simulink model "HW7_simulink"  (R2021b)
settings: Solver=ode4  StartTime=0.0  StopTime=5  FixedStep=.005  RelTol=1e-3
values from neighbouring files (symbols this model uses):
  A = [1 0; 3 -1]    [HW2.m]    (also in HW5.m = [0 -1; 1 -1]; HW6.m = [-1 0; 0 -2]; HW7.m = double(subs(A_sym,[x1;x2;x3;x4;u],[x_star;u_star])))
  B = [1; 0]    [HW5.m]    (also in HW6.m = [1; 3]; HW7.m = double(subs(B_sym,[x1;x2;x3;x4;u],[x_star;u_star])))
  C = eye(2)    [HW5.m]    (also in HW7.m = [1 0 0 0;0 0 1 0])
  D = zeros(2,1)    [HW5.m]    (also in HW7.m)
  g = 10    [HW7.m]
  K = round(time/Ts)    [HW5.m]    (also in HW7.m = acker(A,B,s_desired))
  L = place(A',C',s_obs_desired)'    [HW7.m]
  l = 1    [HW7.m]
  m = 1    [HW7.m]
  M = [4 2 1; 4 -2 1; 4 1 0]    [HW2.m]    (also in HW7.m = 10)
undefined symbols (not defined in the file or in its folder): magnitude
settings Model: Creator=17165  LastModifiedBy=17165

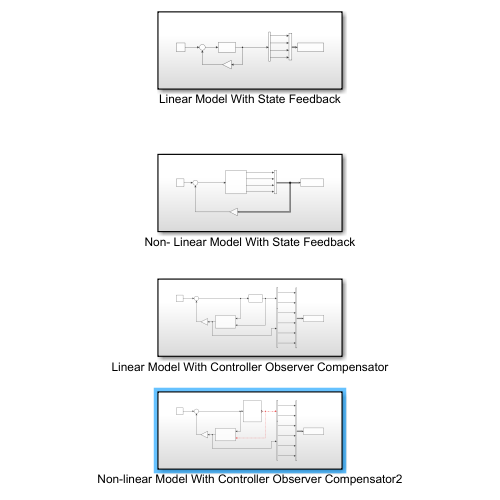
[thumbnail: Simulink's stored preview of the top-level diagram]
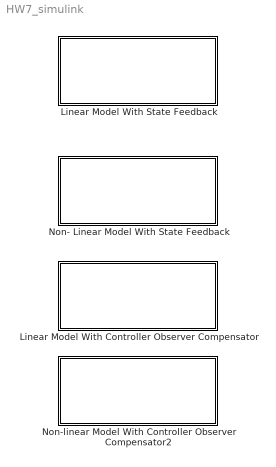
== system HW7_simulink ==
  Linear Model With Controller Observer Compensator : Subsystem
  Linear Model With State Feedback : Subsystem
  Non- Linear Model With State Feedback : Subsystem
  Non-linear Model With Controller Observer Compensator2 : Subsystem

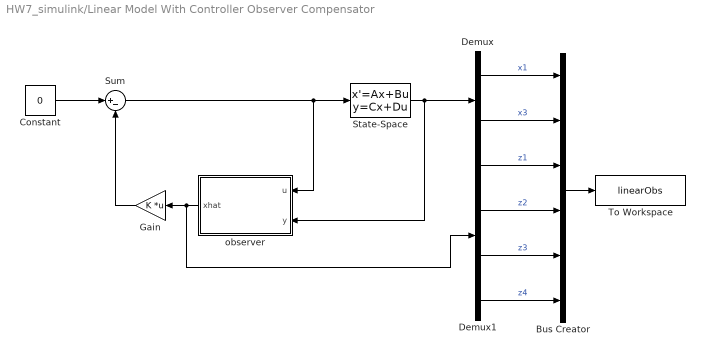
== system HW7_simulink/Linear Model With Controller Observer Compensator ==
  Bus Creator : BusCreator  Inputs=6
  Constant : Constant  Value=0
  Demux : Demux  Outputs=2
  Demux1 : Demux
  Gain : Gain  Gain=K  Multiplication=Matrix(K*u)
  State-Space : StateSpace  A=A  B=B  C=C  D=D  InitialCondition=[-2 3 -1 2]
  Sum : Sum  Inputs=|+-
  To Workspace : ToWorkspace  VariableName=linearObs  SaveFormat=Structure With Time  SampleTime=-1
  observer : Subsystem
  wires:
  State-Space/1 -> observer/2(y), Demux/1
  Constant/1 -> Sum/1
  Gain/1 -> Sum/2
  Sum/1 -> observer/1(u), State-Space/1
  Demux/1 -> Bus Creator/1  "x1"
  Demux/2 -> Bus Creator/2  "x3"
  Bus Creator/1 -> To Workspace/1
  observer/1(xhat) -> Demux1/1, Gain/1
  Demux1/1 -> Bus Creator/3  "z1"
  Demux1/2 -> Bus Creator/4  "z2"
  Demux1/3 -> Bus Creator/5  "z3"
  Demux1/4 -> Bus Creator/6  "z4"

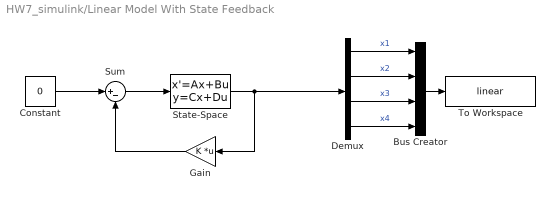
== system HW7_simulink/Linear Model With State Feedback ==
  Bus Creator : BusCreator  Inputs=4
  Constant : Constant  Value=0
  Demux : Demux
  Gain : Gain  Gain=K  Multiplication=Matrix(K*u)
  State-Space : StateSpace  A=A  B=B  C=eye(4)  D=zeros(4,1)  InitialCondition=[-2 3 -1 2]
  Sum : Sum  Inputs=|+-
  To Workspace : ToWorkspace  VariableName=linear  SaveFormat=Structure With Time  SampleTime=-1
  wires:
  State-Space/1 -> Gain/1, Demux/1
  Constant/1 -> Sum/1
  Gain/1 -> Sum/2
  Sum/1 -> State-Space/1
  Demux/1 -> Bus Creator/1  "x1"
  Demux/2 -> Bus Creator/2  "x2"
  Demux/3 -> Bus Creator/3  "x3"
  Demux/4 -> Bus Creator/4  "x4"
  Bus Creator/1 -> To Workspace/1

== system HW7_simulink/Non- Linear Model With State Feedback ==
  Bus Creator : BusCreator  Inputs=4
  Constant : Constant  Value=0
  Gain : Gain  Gain=K  Multiplication=Matrix(K*u)
  Subsystem : Subsystem
      mask Display: disp('Non-linear Model')
  Sum : Sum  Inputs=|+-
  To Workspace : ToWorkspace  VariableName=nonlinear  SaveFormat=Structure With Time  SampleTime=-1
  wires:
  Constant/1 -> Sum/1
  Gain/1 -> Sum/2
  Sum/1 -> Subsystem/1(u)
  Subsystem/1(x1) -> Bus Creator/1  "x1"
  Subsystem/2(x2) -> Bus Creator/2  "x2"
  Subsystem/3(x3) -> Bus Creator/3  "x3"
  Subsystem/4(x4) -> Bus Creator/4  "x4"
  Bus Creator/1 -> Gain/1, To Workspace/1

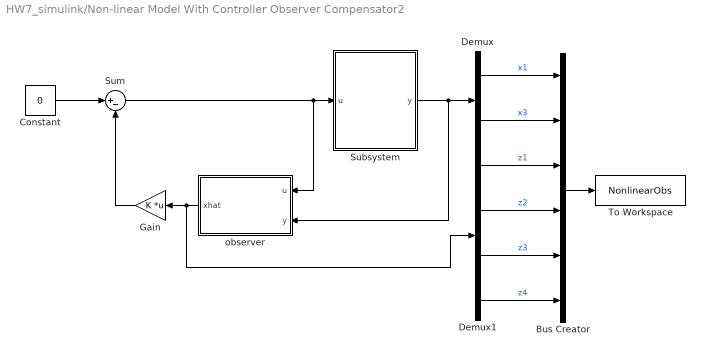
== system HW7_simulink/Non-linear Model With Controller Observer Compensator2 ==
  Bus Creator : BusCreator  Inputs=6
  Constant : Constant  Value=0
  Demux : Demux  Outputs=2
  Demux1 : Demux
  Gain : Gain  Gain=K  Multiplication=Matrix(K*u)
  Subsystem : Subsystem
      mask Display: disp('Non-linear Model')
  Sum : Sum  Inputs=|+-
  To Workspace : ToWorkspace  VariableName=NonlinearObs  SaveFormat=Structure With Time  SampleTime=-1
  observer : Subsystem
  wires:
  Demux1/4 -> Bus Creator/6  "z4"
  Demux1/3 -> Bus Creator/5  "z3"
  Demux1/2 -> Bus Creator/4  "z2"
  Demux1/1 -> Bus Creator/3  "z1"
  observer/1(xhat) -> Gain/1, Demux1/1
  Bus Creator/1 -> To Workspace/1
  Demux/2 -> Bus Creator/2  "x3"
  Demux/1 -> Bus Creator/1  "x1"
  Sum/1 -> observer/1(u), Subsystem/1(u)
  Gain/1 -> Sum/2
  Constant/1 -> Sum/1
  Subsystem/1(y) -> Demux/1, observer/2(y)

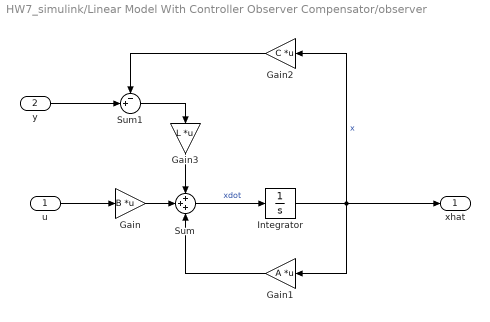
== system HW7_simulink/Linear Model With Controller Observer Compensator/observer ==
  u : Inport
  y : Inport  Port=2
  Gain : Gain  Gain=B  Multiplication=Matrix(K*u)
  Gain1 : Gain  Gain=A  Multiplication=Matrix(K*u)
  Gain2 : Gain  Gain=C  Multiplication=Matrix(K*u)
  Gain3 : Gain  Gain=L  Multiplication=Matrix(K*u)
  Integrator : Integrator
  Sum : Sum  Inputs=+++
  Sum1 : Sum  Inputs=-+|
  xhat : Outport
  wires:
  u/1 -> Gain/1
  Integrator/1 -> Gain2/1, Gain1/1, xhat/1  "x"
  Sum/1 -> Integrator/1  "xdot"
  Gain/1 -> Sum/2
  Gain1/1 -> Sum/3
  y/1 -> Sum1/2
  Gain2/1 -> Sum1/1
  Sum1/1 -> Gain3/1
  Gain3/1 -> Sum/1

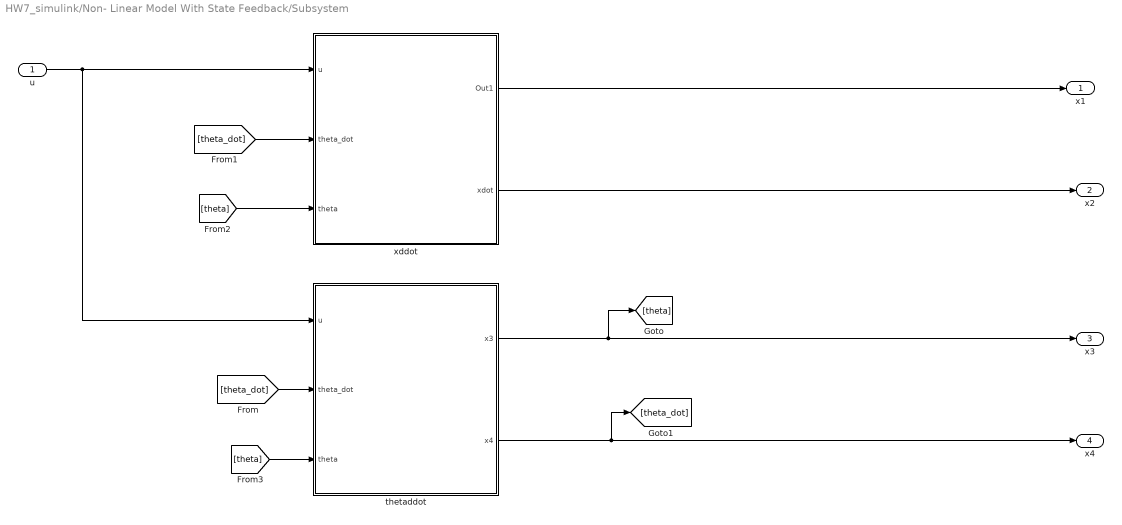
== system HW7_simulink/Non- Linear Model With State Feedback/Subsystem ==
  u : Inport
  thetaddot : Subsystem
  "xddot " : Subsystem
  x1 : Outport
  x2 : Outport  Port=2
  x3 : Outport  Port=3
  x4 : Outport  Port=4
  wires:
  u/1 -> thetaddot/1(u), "xddot "/1(u)
  "xddot "/1(Out1) -> x1/1
  "xddot "/2(xdot) -> x2/1
  thetaddot/1(x3) -> [theta], x3/1
  thetaddot/2(x4) -> [theta_dot], x4/1
  [theta_dot] -> thetaddot/2(theta_dot)
  [theta_dot] -> "xddot "/2(theta_dot)
  [theta] -> "xddot "/3(theta)
  [theta] -> thetaddot/3(theta)

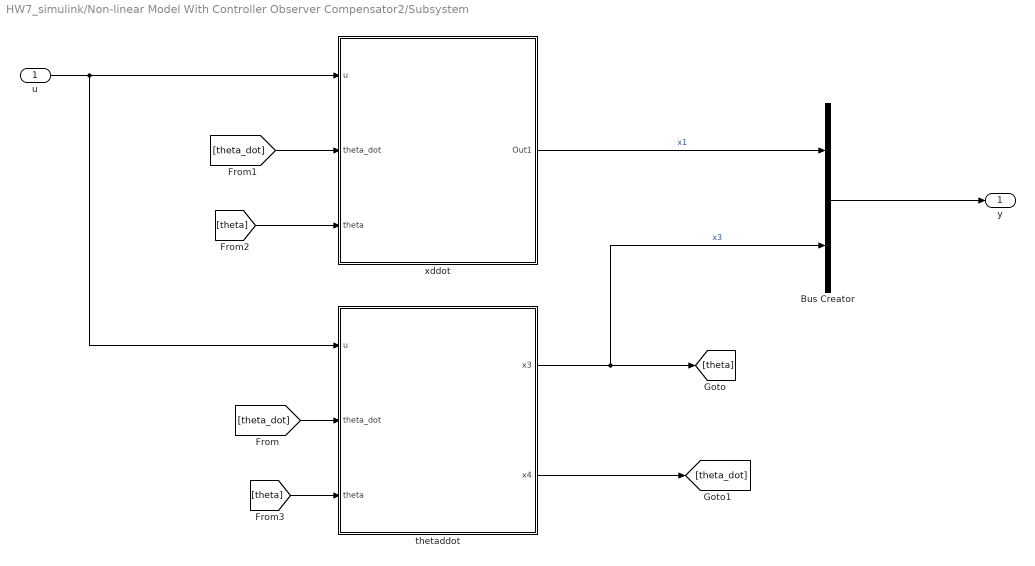
== system HW7_simulink/Non-linear Model With Controller Observer Compensator2/Subsystem ==
  u : Inport
  Bus Creator : BusCreator  Inputs=2
  thetaddot : Subsystem
  "xddot " : Subsystem
  y : Outport
  wires:
  u/1 -> thetaddot/1(u), "xddot "/1(u)
  thetaddot/2(x4) -> [theta_dot]
  [theta_dot] -> thetaddot/2(theta_dot)
  [theta_dot] -> "xddot "/2(theta_dot)
  [theta] -> "xddot "/3(theta)
  [theta] -> thetaddot/3(theta)
  Bus Creator/1 -> y/1
  thetaddot/1(x3) -> Bus Creator/2, [theta]  "x3"
  "xddot "/1(Out1) -> Bus Creator/1  "x1"

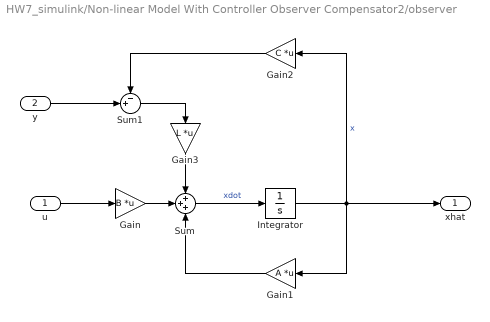
== system HW7_simulink/Non-linear Model With Controller Observer Compensator2/observer ==
  u : Inport
  y : Inport  Port=2
  Gain : Gain  Gain=B  Multiplication=Matrix(K*u)
  Gain1 : Gain  Gain=A  Multiplication=Matrix(K*u)
  Gain2 : Gain  Gain=C  Multiplication=Matrix(K*u)
  Gain3 : Gain  Gain=L  Multiplication=Matrix(K*u)
  Integrator : Integrator
  Sum : Sum  Inputs=+++
  Sum1 : Sum  Inputs=-+|
  xhat : Outport
  wires:
  Gain3/1 -> Sum/1
  Sum1/1 -> Gain3/1
  Gain2/1 -> Sum1/1
  y/1 -> Sum1/2
  Gain1/1 -> Sum/3
  Gain/1 -> Sum/2
  Sum/1 -> Integrator/1  "xdot"
  Integrator/1 -> xhat/1, Gain1/1, Gain2/1  "x"
  u/1 -> Gain/1

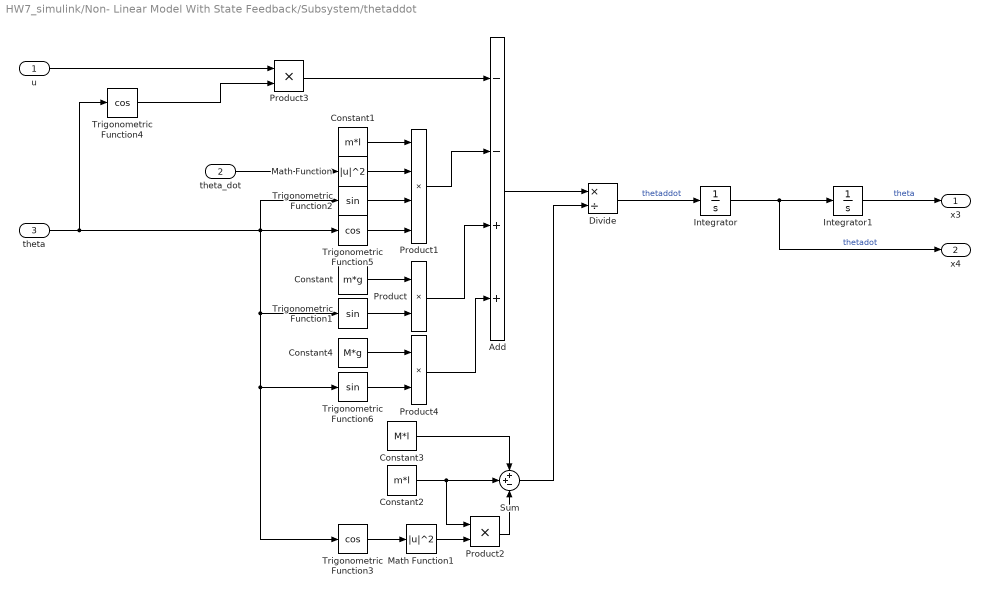
== system HW7_simulink/Non- Linear Model With State Feedback/Subsystem/thetaddot ==
  u : Inport
  theta_dot : Inport  Port=2
  theta : Inport  Port=3
  Add : Sum  Inputs=--++
  Constant : Constant  Value=m*g
  Constant1 : Constant  Value=m*l
  Constant2 : Constant  Value=m*l
  Constant3 : Constant  Value=M*l
  Constant4 : Constant  Value=M*g
  Divide : Product  Inputs=*/
  Integrator : Integrator  InitialCondition=2
  Integrator1 : Integrator  InitialCondition=-1
  Math Function : Math  Operator=magnitude^2  SaturateOnIntegerOverflow=on
  Math Function1 : Math  Operator=magnitude^2  SaturateOnIntegerOverflow=on
  Product{,2..4} (4 alike) : Product
  Product1 : Product  Inputs=4
  Sum : Sum  Inputs=++-
  Trigonometric Function1 : Trigonometry
  Trigonometric Function2 : Trigonometry
  Trigonometric Function3 : Trigonometry  Operator=cos
  Trigonometric Function4 : Trigonometry  Operator=cos
  Trigonometric Function5 : Trigonometry  Operator=cos
  Trigonometric Function6 : Trigonometry
  x3 : Outport
  x4 : Outport  Port=2
  wires:
  Integrator/1 -> x4/1, Integrator1/1  "thetadot"
  Trigonometric Function2/1 -> Product1/3
  Product1/1 -> Add/2
  theta_dot/1 -> Math Function/1
  Product/1 -> Add/3
  Trigonometric Function1/1 -> Product/2
  Constant/1 -> Product/1
  Math Function/1 -> Product1/2
  Integrator1/1 -> x3/1  "theta"
  Constant1/1 -> Product1/1
  Add/1 -> Divide/1
  Divide/1 -> Integrator/1  "thetaddot"
  Constant2/1 -> Product2/1, Sum/2
  Constant3/1 -> Sum/1
  Trigonometric Function3/1 -> Math Function1/1
  Math Function1/1 -> Product2/2
  Product2/1 -> Sum/3
  Sum/1 -> Divide/2
  u/1 -> Product3/1
  Trigonometric Function4/1 -> Product3/2
  Product3/1 -> Add/1
  Trigonometric Function5/1 -> Product1/4
  Constant4/1 -> Product4/1
  theta/1 -> Trigonometric Function4/1, Trigonometric Function2/1, Trigonometric Function5/1, Trigonometric Function6/1, Trigonometric Function3/1, Trigonometric Function1/1
  Product4/1 -> Add/4
  Trigonometric Function6/1 -> Product4/2

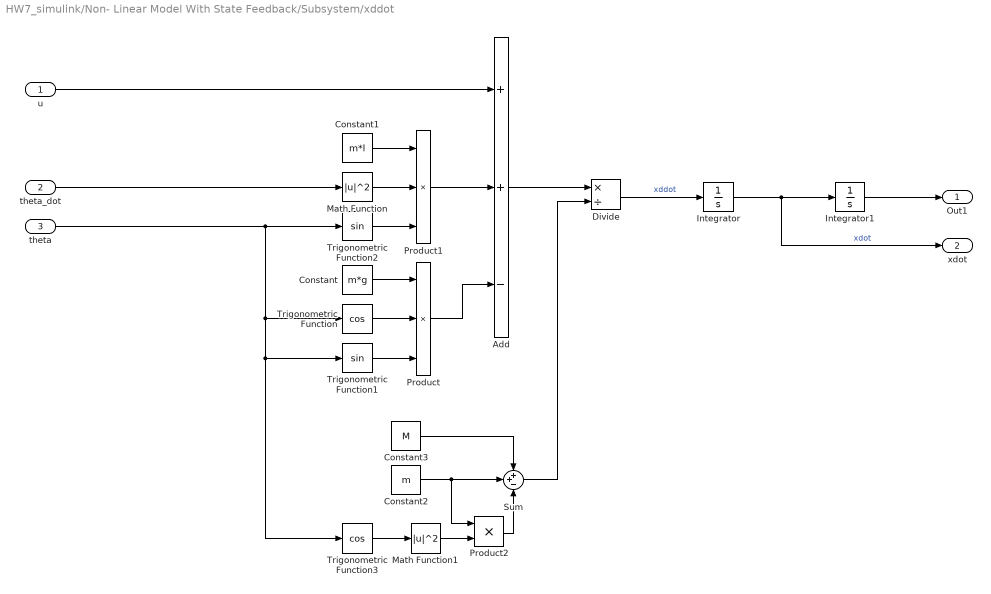
== system HW7_simulink/Non- Linear Model With State Feedback/Subsystem/xddot  ==
  u : Inport
  theta_dot : Inport  Port=2
  theta : Inport  Port=3
  Add : Sum  Inputs=++-
  Constant : Constant  Value=m*g
  Constant1 : Constant  Value=m*l
  Constant2 : Constant  Value=m
  Constant3 : Constant  Value=M
  Divide : Product  Inputs=*/
  Integrator : Integrator  InitialCondition=3
  Integrator1 : Integrator  InitialCondition=-2
  Math Function : Math  Operator=magnitude^2  SaturateOnIntegerOverflow=on
  Math Function1 : Math  Operator=magnitude^2  SaturateOnIntegerOverflow=on
  Product : Product  Inputs=3
  Product1 : Product  Inputs=3
  Product2 : Product
  Sum : Sum  Inputs=++-
  Trigonometric Function : Trigonometry  Operator=cos
  Trigonometric Function1 : Trigonometry
  Trigonometric Function2 : Trigonometry
  Trigonometric Function3 : Trigonometry  Operator=cos
  Out1 : Outport
  xdot : Outport  Port=2
  wires:
  theta/1 -> Trigonometric Function3/1, Trigonometric Function1/1, Trigonometric Function/1, Trigonometric Function2/1
  Integrator/1 -> xdot/1, Integrator1/1  "xdot"
  Trigonometric Function2/1 -> Product1/3
  Product1/1 -> Add/2
  theta_dot/1 -> Math Function/1
  Product/1 -> Add/3
  Trigonometric Function1/1 -> Product/3
  Constant/1 -> Product/1
  Math Function/1 -> Product1/2
  Trigonometric Function/1 -> Product/2
  Integrator1/1 -> Out1/1
  Constant1/1 -> Product1/1
  u/1 -> Add/1
  Add/1 -> Divide/1
  Divide/1 -> Integrator/1  "xddot"
  Constant2/1 -> Product2/1, Sum/2
  Constant3/1 -> Sum/1
  Trigonometric Function3/1 -> Math Function1/1
  Math Function1/1 -> Product2/2
  Product2/1 -> Sum/3
  Sum/1 -> Divide/2

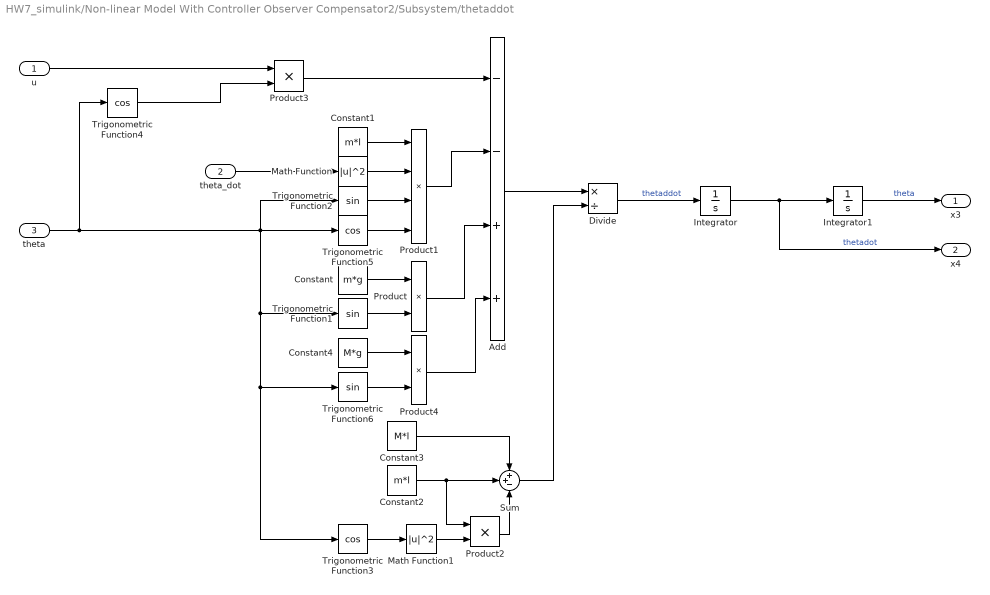
== system HW7_simulink/Non-linear Model With Controller Observer Compensator2/Subsystem/thetaddot ==
  u : Inport
  theta_dot : Inport  Port=2
  theta : Inport  Port=3
  Add : Sum  Inputs=--++
  Constant : Constant  Value=m*g
  Constant1 : Constant  Value=m*l
  Constant2 : Constant  Value=m*l
  Constant3 : Constant  Value=M*l
  Constant4 : Constant  Value=M*g
  Divide : Product  Inputs=*/
  Integrator : Integrator  InitialCondition=.2
  Integrator1 : Integrator  InitialCondition=-.1
  Math Function : Math  Operator=magnitude^2  SaturateOnIntegerOverflow=on
  Math Function1 : Math  Operator=magnitude^2  SaturateOnIntegerOverflow=on
  Product{,2..4} (4 alike) : Product
  Product1 : Product  Inputs=4
  Sum : Sum  Inputs=++-
  Trigonometric Function1 : Trigonometry
  Trigonometric Function2 : Trigonometry
  Trigonometric Function3 : Trigonometry  Operator=cos
  Trigonometric Function4 : Trigonometry  Operator=cos
  Trigonometric Function5 : Trigonometry  Operator=cos
  Trigonometric Function6 : Trigonometry
  x3 : Outport
  x4 : Outport  Port=2
  wires:
  Integrator/1 -> x4/1, Integrator1/1  "thetadot"
  Trigonometric Function2/1 -> Product1/3
  Product1/1 -> Add/2
  theta_dot/1 -> Math Function/1
  Product/1 -> Add/3
  Trigonometric Function1/1 -> Product/2
  Constant/1 -> Product/1
  Math Function/1 -> Product1/2
  Integrator1/1 -> x3/1  "theta"
  Constant1/1 -> Product1/1
  Add/1 -> Divide/1
  Divide/1 -> Integrator/1  "thetaddot"
  Constant2/1 -> Product2/1, Sum/2
  Constant3/1 -> Sum/1
  Trigonometric Function3/1 -> Math Function1/1
  Math Function1/1 -> Product2/2
  Product2/1 -> Sum/3
  Sum/1 -> Divide/2
  u/1 -> Product3/1
  Trigonometric Function4/1 -> Product3/2
  Product3/1 -> Add/1
  Trigonometric Function5/1 -> Product1/4
  Constant4/1 -> Product4/1
  theta/1 -> Trigonometric Function4/1, Trigonometric Function2/1, Trigonometric Function5/1, Trigonometric Function6/1, Trigonometric Function3/1, Trigonometric Function1/1
  Product4/1 -> Add/4
  Trigonometric Function6/1 -> Product4/2

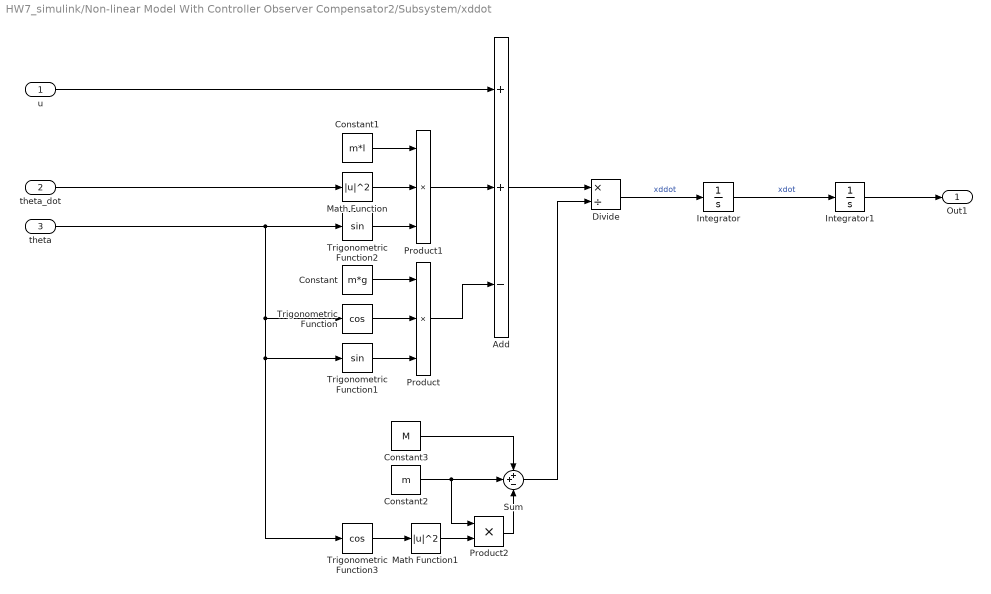
== system HW7_simulink/Non-linear Model With Controller Observer Compensator2/Subsystem/xddot  ==
  u : Inport
  theta_dot : Inport  Port=2
  theta : Inport  Port=3
  Add : Sum  Inputs=++-
  Constant : Constant  Value=m*g
  Constant1 : Constant  Value=m*l
  Constant2 : Constant  Value=m
  Constant3 : Constant  Value=M
  Divide : Product  Inputs=*/
  Integrator : Integrator  InitialCondition=.3
  Integrator1 : Integrator  InitialCondition=-.2
  Math Function : Math  Operator=magnitude^2  SaturateOnIntegerOverflow=on
  Math Function1 : Math  Operator=magnitude^2  SaturateOnIntegerOverflow=on
  Product : Product  Inputs=3
  Product1 : Product  Inputs=3
  Product2 : Product
  Sum : Sum  Inputs=++-
  Trigonometric Function : Trigonometry  Operator=cos
  Trigonometric Function1 : Trigonometry
  Trigonometric Function2 : Trigonometry
  Trigonometric Function3 : Trigonometry  Operator=cos
  Out1 : Outport
  wires:
  theta/1 -> Trigonometric Function3/1, Trigonometric Function1/1, Trigonometric Function/1, Trigonometric Function2/1
  Integrator/1 -> Integrator1/1  "xdot"
  Trigonometric Function2/1 -> Product1/3
  Product1/1 -> Add/2
  theta_dot/1 -> Math Function/1
  Product/1 -> Add/3
  Trigonometric Function1/1 -> Product/3
  Constant/1 -> Product/1
  Math Function/1 -> Product1/2
  Trigonometric Function/1 -> Product/2
  Integrator1/1 -> Out1/1
  Constant1/1 -> Product1/1
  u/1 -> Add/1
  Add/1 -> Divide/1
  Divide/1 -> Integrator/1  "xddot"
  Constant2/1 -> Product2/1, Sum/2
  Constant3/1 -> Sum/1
  Trigonometric Function3/1 -> Math Function1/1
  Math Function1/1 -> Product2/2
  Product2/1 -> Sum/3
  Sum/1 -> Divide/2
